simulink model "lab6_2017a"  (R2017a)
settings: Solver=FixedStepDiscrete  StartTime=0.0  StopTime=inf  FixedStep=mdl_T_sample  RelTol=1e-3
values from neighbouring files (symbols this model uses):
  mdl_byte1 = mdl.byte1    [lab6.m]    (also in lab6_rt.m)
libraries: arduinolib x5, svdutilitieslib x3, MinSegLibrary_M2V3 x2, simulink x1
settings Model: SimulationMode=external  ExtModeTrigDuration=2  Creator=kando  LastModifiedBy=kando
settings DataIOCC: SaveOutput=off  SignalLogging=off  DSMLogging=off  VisualizeSimOutput=off  SaveTime=off
settings OptimizationCC: LifeSpan=Inf  MaxStackSize=64  SimCompilerOptimization=on  AccelVerboseBuild=on
settings DebuggingCC: AllowSymbolicDim=off  SFUnexpectedBacktrackingDiag=warning  SFNoUnconditionalDefaultTransitionDiag=warning  SFExecutionAtInitializationDiag=none
settings HardwareCC: ProdBitPerInt=16  ProdBitPerPointer=16  ProdBitPerSizeT=16  ProdBitPerPtrDiffT=16  ProdLargestAtomicFloat=None  ProdWordSize=8  ProdHWDeviceType=Atmel->AVR  UseEmbeddedCoderFeatures=off  UseSimulinkCoderFeatures=off
settings ModelReferenceCC: PropagateSignalLabelsOutOfModel=off
settings SFSimCC: MATLABDynamicMemAlloc=off
settings RTWCC: SystemTargetFile=ert.tlc  HardwareBoard=Arduino Mega 2560  TLCOptions=-aInlineSetEventsForThisBaseRateFcn=TLC_FALSE -aSuppressMultiTaskScheduler=TLC_FALSE -aRateBasedStepFcn=1  TemplateMakefile=ert_default_tmf  Description=Embedded Coder  Toolchain=Arduino AVR  BuildConfiguration=Faster Runs
settings CodeAppCC: MangleLength=10
settings ERTTargetCC: MultiwordLength=2048  ERTCustomFileBanners=off  SupportContinuousTime=on  SupportNonInlinedSFcns=on  RemoveResetFunc=off  SupportVariableSizeSignals=on  ModelStepFunctionPrototypeControlCompliant=off  ConvertIfToSwitch=off  SuppressUnreachableDefaultCases=off
settings ConfigComp: CovMetricSettings=dw  CovHtmlReporting=on  CovSaveCumulativeToWorkspaceVar=on  CovSaveSingleToWorkspaceVar=on  CovExternalEMLEnable=off

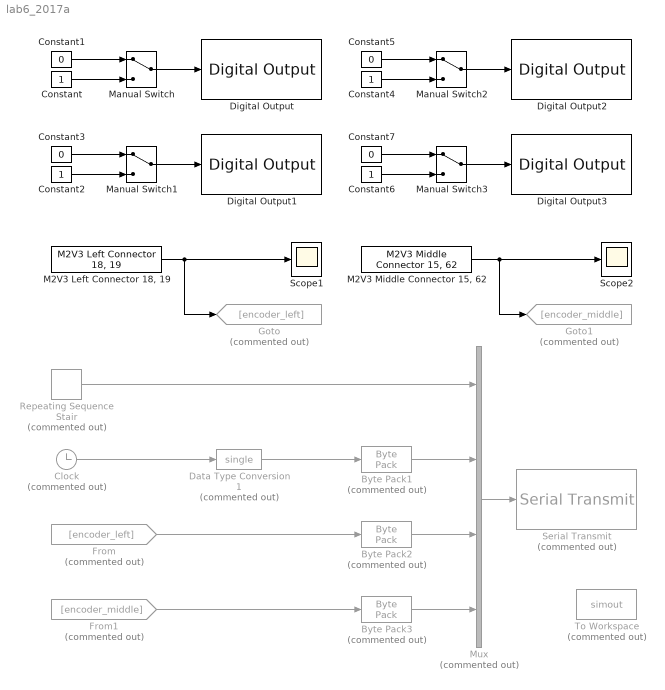
== system lab6_2017a ==
  Byte Pack1 : svdutilitieslib/Byte Pack  Commented=on  datatypes={'single'}  byteAlign=1  blockPlatform=arduinoert
      settings: SourceProductName=Simulink Support Package for Arduino Hardware
  Byte Pack2 : svdutilitieslib/Byte Pack  Commented=on  datatypes={'int32'}  byteAlign=1  blockPlatform=arduinoert
      settings: SourceProductName=Simulink Support Package for Arduino Hardware
  Byte Pack3 : svdutilitieslib/Byte Pack  Commented=on  datatypes={'int32'}  byteAlign=1  blockPlatform=arduinoert
      settings: SourceProductName=Simulink Support Package for Arduino Hardware
  Clock : Clock  Commented=on
      settings: Decimation=round( 1 / mdl_T_sample )
  Constant{,2,4,6} (4 alike) : Constant
  Constant{1,3,5,7} (4 alike) : Constant  Value=0
  Data Type Conversion1 : DataTypeConversion  Commented=on  OutDataTypeStr=single
  Digital Output : arduinolib/Digital Output  pinNumber=2  blockPlatform=arduino
  Digital Output1 : arduinolib/Digital Output  pinNumber=5  blockPlatform=arduino
  Digital Output2 : arduinolib/Digital Output  pinNumber=6  blockPlatform=arduino
  Digital Output3 : arduinolib/Digital Output  pinNumber=8  blockPlatform=arduino
  From : From  Commented=on  GotoTag=encoder_left
  From1 : From  Commented=on  GotoTag=encoder_middle
  Goto : Goto  Commented=on  GotoTag=encoder_left
  Goto1 : Goto  Commented=on  GotoTag=encoder_middle
  "M2V3 Left Connector 18, 19" : MinSegLibrary_M2V3/M2V3 Left Connector 18, 19  Encoder=1  PinA=19  PinB=18  PWMFSelect=3  PWMTimer=-1
      settings: SourceProductName=Rensselaer Arduino Support Package
  "M2V3 Middle Connector 15, 62" : MinSegLibrary_M2V3/M2V3 Middle Connector 15, 62  Encoder=3  PinA=15  PinB=62  PWMFSelect=3  PWMTimer=-1
      settings: SourceProductName=Rensselaer Arduino Support Package
  Manual Switch{,1..3} (4 alike) : ManualSwitch
  Mux : Mux  Commented=on
  Repeating Sequence Stair : simulink/Sources/Repeating Sequence Stair  Commented=on  OutValues=1%mdl_byte1  tsamp=-1  OutMin=[]  OutMax=[]  OutDataTypeStr=uint8  OutputDataTypeScalingMode=uint8  OutDataType=fixdt(0,8)  ConRadixGroup=Best Precision: Vector-wise  OutScaling=2^-12
  Scope1 : Scope
  Scope2 : Scope
  Serial Transmit : arduinolib/Serial Transmit  Commented=on  portNumber=0  sendmode=write  sendformat=Decimal  floatprecision=2  blockPlatform=arduino
      settings: SourceProductName=Simulink Support Package for Arduino Hardware
  To Workspace : ToWorkspace  Commented=on  VariableName=simout  SaveFormat=Timeseries  SampleTime=-1
  wires:
  Constant/1 -> Manual Switch/2
  Constant1/1 -> Manual Switch/1
  Manual Switch/1 -> Digital Output/1
  Manual Switch1/1 -> Digital Output1/1
  Constant3/1 -> Manual Switch1/1
  Constant2/1 -> Manual Switch1/2
  Constant7/1 -> Manual Switch3/1
  Constant5/1 -> Manual Switch2/1
  Manual Switch3/1 -> Digital Output3/1
  Constant4/1 -> Manual Switch2/2
  Manual Switch2/1 -> Digital Output2/1
  Constant6/1 -> Manual Switch3/2
  "M2V3 Middle Connector 15, 62"/1 -> Goto1/1, Scope2/1
  "M2V3 Left Connector 18, 19"/1 -> Goto/1, Scope1/1
  Mux/1 -> Serial Transmit/1
  Repeating Sequence Stair/1 -> Mux/1
  From/1 -> Byte Pack2/1
  From1/1 -> Byte Pack3/1
  Clock/1 -> Data Type Conversion1/1
  Data Type Conversion1/1 -> Byte Pack1/1
  Byte Pack1/1 -> Mux/2
  Byte Pack2/1 -> Mux/3
  Byte Pack3/1 -> Mux/4
